simulink subsystem "Plant_Attitude"  (R2025a)
settings: Solver=VariableStepAuto  StartTime=0.0  StopTime=10.0  RelTol=1e-3
undefined symbols (not defined in the file): config
libraries: matrix_library x1, aerolibutil x1
settings Model: Creator=Jackt  LastModifiedBy=Jackt

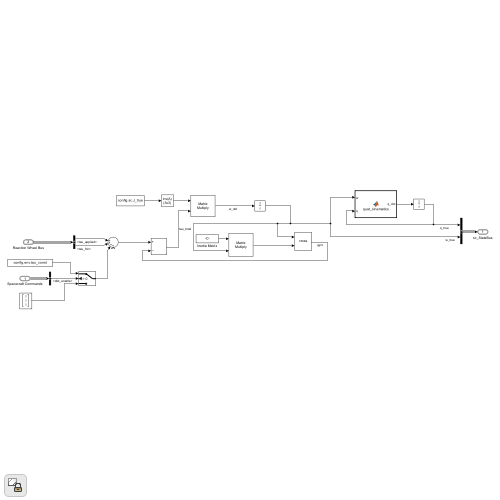
[thumbnail: Simulink's stored preview of the top-level diagram]
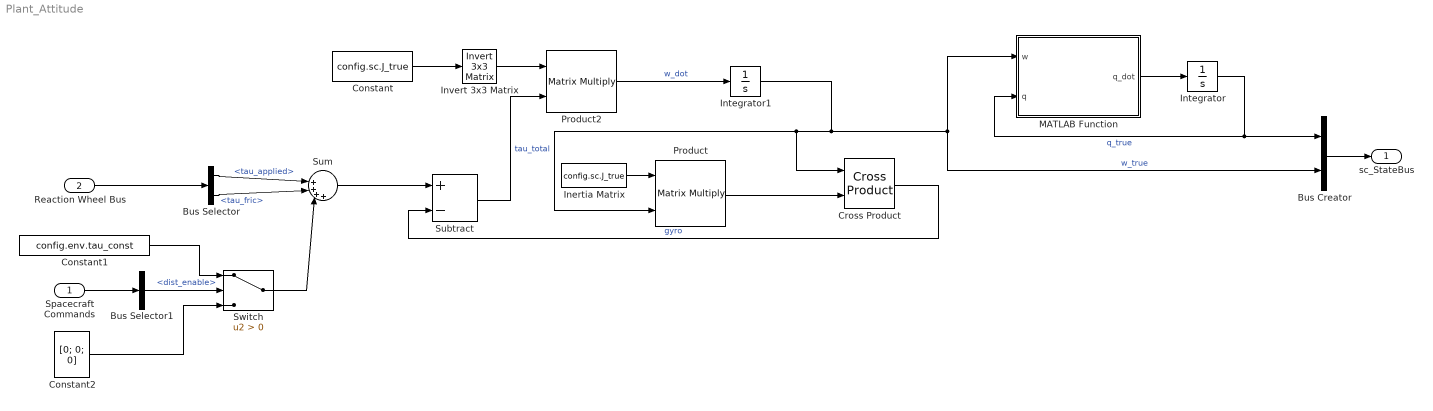
== system Plant_Attitude ==
  Spacecraft Commands : Inport  OutDataTypeStr=Bus: commandBus
  Reaction Wheel Bus : Inport  Port=2  OutDataTypeStr=Bus: reactionWheelBus
  Bus Creator : BusCreator  Inputs=2  OutDataTypeStr=Bus: sc_stateBus
  Bus Selector : BusSelector  OutputSignals=tau_applied,tau_fric
  Bus Selector1 : BusSelector  OutputSignals=dist_enable
  Constant : Constant  Value=config.sc.J_true  VectorParams1D=off
  Constant1 : Constant  Value=config.env.tau_const  VectorParams1D=off
  Constant2 : Constant  Value=[0; 0; 0]  VectorParams1D=off
  Cross Product : matrix_library/Cross Product
  Inertia Matrix : Constant  Value=config.sc.J_true  VectorParams1D=off
  Integrator : Integrator  InitialCondition=config.ic.q_0
  Integrator1 : Integrator  InitialCondition=config.ic.w_0
  Invert 3x3 Matrix : aerolibutil/Invert  3x3 Matrix
  MATLAB Function : MATLAB Function  TreatAsAtomicUnit=on
  Product : Product  Multiplication=Matrix(*)
  Product2 : Product  Multiplication=Matrix(*)
  Subtract : Sum  Inputs=+-
  Sum : Sum  Inputs=||++++
  Switch : Switch  Criteria=u2 > Threshold  SaturateOnIntegerOverflow=off  InputSameDT=off
  sc_StateBus : Outport  OutDataTypeStr=Bus: sc_stateBus
  wires:
  Inertia Matrix/1 -> Product/1
  Subtract/1 -> Product2/2  "tau_total"
  Sum/1 -> Subtract/1
  Bus Selector/1 -> Sum/1  "<tau_applied>"
  Invert 3x3 Matrix/1 -> Product2/1
  Product2/1 -> Integrator1/1  "w_dot"
  Integrator1/1 -> MATLAB Function/1(w), Bus Creator/2, Product/2, Cross Product/1  "w_true"
  Cross Product/1 -> Subtract/2  "gyro"
  MATLAB Function/1(q_dot) -> Integrator/1
  Product/1 -> Cross Product/2
  Integrator/1 -> Bus Creator/1, MATLAB Function/2(q)  "q_true"
  Constant/1 -> Invert 3x3 Matrix/1
  Bus Selector/2 -> Sum/2  "<tau_fric>"
  Bus Creator/1 -> sc_StateBus/1
  Reaction Wheel Bus/1 -> Bus Selector/1
  Spacecraft Commands/1 -> Bus Selector1/1
  Bus Selector1/1 -> Switch/2  "<dist_enable>"
  Constant1/1 -> Switch/1
  Constant2/1 -> Switch/3
  Switch/1 -> Sum/3

== matlab function Plant_Attitude/MATLAB Function ==
  data: w input; q_dot output size=[4 1]; q input
function q_dot = quat_kinematics(w, q)
% q is scalar-first [q0;q1;q2;q3], w = [wx;wy;wz]
wx = w(1); wy = w(2); wz = w(3);

Omega = [ 0   -wx  -wy  -wz;
          wx   0    wz  -wy;
          wy  -wz   0    wx;
          wz   wy  -wx   0 ];

q_dot = 0.5 * Omega * q;
end
